simulink model "TASK7_kalman_filter"  (R2023b)
settings: Solver=VariableStepAuto  StartTime=0.0  StopTime=10  MaxStep=0.01  RelTol=1e-3  EnableMultiTasking=on
values from neighbouring files (symbols this model uses):
  b = 0.2    [TASK0_main_code.m]
  dphi0 = 0.1    [TASK0_main_code.m]
  dx0 = 0.01    [TASK0_main_code.m]
  g = 9.81    [TASK0_main_code.m]
  J_s = 1/3*m*l^2    (= 4.99725166667)    [TASK0_main_code.m]
  K = place(A_lin, B_lin, p)    [TASK0_main_code.m]
  KF = ss(A_lin-L*C_lin(2,:), [B_lin L], eye(4), 0*[B_lin L])    [TASK0_main_code.m]
  l = 3.11    [TASK0_main_code.m]
  m = 1.55    [TASK0_main_code.m]
  M = 7.87    [TASK0_main_code.m]
  noise_mean = 0    [TASK0_main_code.m]
  noise_sample_time = 0.001    [TASK0_main_code.m]
  noise_seed = 10000    [TASK0_main_code.m]
  phi0 = 0.05    [TASK0_main_code.m]
  sigma_wd = [ 1 , 0  , 0 , 0 ... (first row only)    [TASK0_main_code.m]
  sigma_wd2 = [ 1 , 0  , 0 , 0 ... (first row only)    [TASK0_main_code.m]
  sigma_wd3 = [ 10 , 0  , 0 , 0 ... (first row only)    [TASK0_main_code.m]
  sigma_wn = 0.1    [TASK0_main_code.m]
  x0 = -0.01    [TASK0_main_code.m]
libraries: dspinverses x3
settings Model: Creator=iklod_000  LastModifiedBy=piri
settings SolverCC: AlgebraicLoopSolver=TrustRegion
settings DataIOCC: ReturnWorkspaceOutputs=off
settings OptimizationCC: LifeSpan=inf
settings DebuggingCC: UnconnectedInputMsg=warning  UnconnectedOutputMsg=warning  UnconnectedLineMsg=warning  SFUnexpectedBacktrackingDiag=warning  SFNoUnconditionalDefaultTransitionDiag=warning  ArithmeticOperatorsInVariantConditions=warning
settings ModelReferenceCC: EnableRefExpFcnMdlSchedulingChecks=on
settings SFSimCC: SimUseLocalCustomCode=off  CustomCodeUndefinedFunction=UseInterfaceOnly
settings RTWCC: RTWUseLocalCustomCode=off
settings CodeAppCC: StateflowObjectComments=on
settings GRTTargetCC: TargetLangStandard=C89/C90 (ANSI)
settings ConfigComp: CovMetricSettings=dw  CovSaveCumulativeToWorkspaceVar=on  CovSaveSingleToWorkspaceVar=on  CovExternalEMLEnable=off

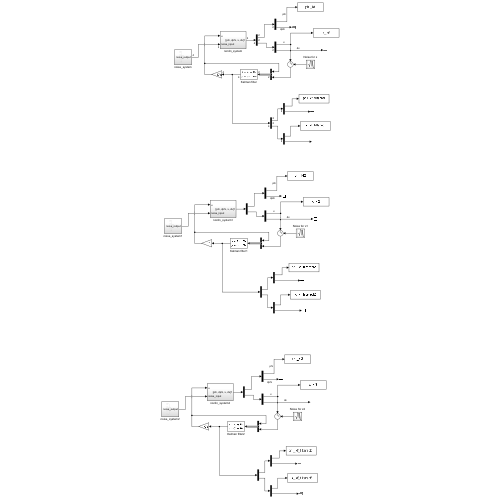
[thumbnail: Simulink's stored preview of the top-level diagram]
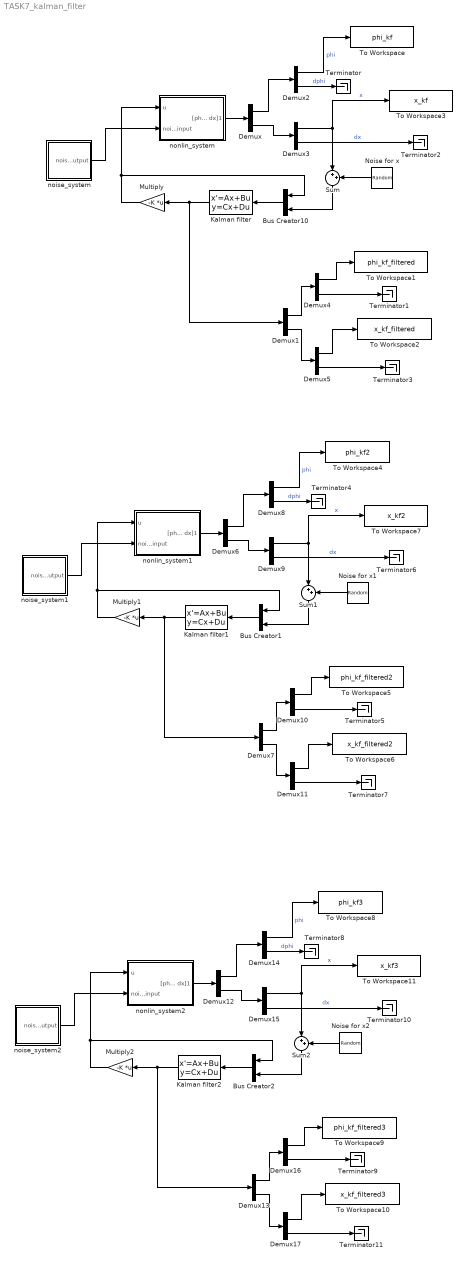
== system TASK7_kalman_filter ==
  Bus Creator1 : BusCreator  Inputs=2
  Bus Creator10 : BusCreator  Inputs=2
  Bus Creator2 : BusCreator  Inputs=2
  Demux{,1..17} (18 alike) : Demux  Outputs=2
  Kalman filter : StateSpace  A=KF.A  B=KF.B  C=KF.C  D=KF.D  InitialCondition=[phi0, dphi0, x0, dx0]
  Kalman filter1 : StateSpace  A=KF.A  B=KF.B  C=KF.C  D=KF.D  InitialCondition=[phi0, dphi0, x0, dx0]
  Kalman filter2 : StateSpace  A=KF.A  B=KF.B  C=KF.C  D=KF.D  InitialCondition=[phi0, dphi0, x0, dx0]
  Multiply : Gain  Gain=-K  Multiplication=Matrix(K*u)
  Multiply1 : Gain  Gain=-K  Multiplication=Matrix(K*u)
  Multiply2 : Gain  Gain=-K  Multiplication=Matrix(K*u)
  Noise for x : RandomNumber  Mean=noise_mean  Variance=sigma_wn  Seed=noise_seed  SampleTime=noise_sample_time
  Noise for x1 : RandomNumber  Mean=noise_mean  Variance=sigma_wn  Seed=noise_seed  SampleTime=noise_sample_time
  Noise for x2 : RandomNumber  Mean=noise_mean  Variance=sigma_wn  Seed=noise_seed  SampleTime=noise_sample_time
  Sum : Sum  Inputs=|++
  Sum1 : Sum  Inputs=|++
  Sum2 : Sum  Inputs=|++
  Terminator{,1..11} (12 alike) : Terminator
  To Workspace : ToWorkspace  VariableName=phi_kf  SaveFormat=Timeseries  SampleTime=-1
  To Workspace1 : ToWorkspace  VariableName=phi_kf_filtered  SaveFormat=Timeseries  SampleTime=-1
  To Workspace10 : ToWorkspace  VariableName=x_kf_filtered3  SaveFormat=Timeseries  SampleTime=-1
  To Workspace11 : ToWorkspace  VariableName=x_kf3  SaveFormat=Timeseries  SampleTime=-1
  To Workspace2 : ToWorkspace  VariableName=x_kf_filtered  SaveFormat=Timeseries  SampleTime=-1
  To Workspace3 : ToWorkspace  VariableName=x_kf  SaveFormat=Timeseries  SampleTime=-1
  To Workspace4 : ToWorkspace  VariableName=phi_kf2  SaveFormat=Timeseries  SampleTime=-1
  To Workspace5 : ToWorkspace  VariableName=phi_kf_filtered2  SaveFormat=Timeseries  SampleTime=-1
  To Workspace6 : ToWorkspace  VariableName=x_kf_filtered2  SaveFormat=Timeseries  SampleTime=-1
  To Workspace7 : ToWorkspace  VariableName=x_kf2  SaveFormat=Timeseries  SampleTime=-1
  To Workspace8 : ToWorkspace  VariableName=phi_kf3  SaveFormat=Timeseries  SampleTime=-1
  To Workspace9 : ToWorkspace  VariableName=phi_kf_filtered3  SaveFormat=Timeseries  SampleTime=-1
  noise_system : Subsystem
  noise_system1 : Subsystem
  noise_system2 : Subsystem
  nonlin_system : Subsystem
  nonlin_system1 : Subsystem
  nonlin_system2 : Subsystem
  wires:
  nonlin_system/1("[phi, dphi, x, dx]1") -> Demux/1
  Demux/1 -> Demux2/1
  Multiply/1 -> Bus Creator10/1, nonlin_system/1(u)
  Demux2/1 -> To Workspace/1  "phi"
  Demux2/2 -> Terminator/1  "dphi"
  Kalman filter/1 -> Demux1/1, Multiply/1
  Demux/2 -> Demux3/1
  Demux3/1 -> To Workspace3/1, Sum/1  "x"
  Noise for x/1 -> Sum/2
  Sum/1 -> Bus Creator10/2
  Bus Creator10/1 -> Kalman filter/1
  Demux3/2 -> Terminator2/1  "dx"
  Demux1/1 -> Demux4/1
  Demux1/2 -> Demux5/1
  Demux4/1 -> To Workspace1/1
  Demux4/2 -> Terminator1/1
  Demux5/1 -> To Workspace2/1
  Demux5/2 -> Terminator3/1
  noise_system/1(noise_output) -> nonlin_system/2(noise_input)
  Sum1/1 -> Bus Creator1/2
  Bus Creator1/1 -> Kalman filter1/1
  Demux9/2 -> Terminator6/1  "dx"
  Kalman filter1/1 -> Demux7/1, Multiply1/1
  Demux10/1 -> To Workspace5/1
  Demux7/2 -> Demux11/1
  Demux11/2 -> Terminator7/1
  Demux6/1 -> Demux8/1
  noise_system1/1(noise_output) -> nonlin_system1/2(noise_input)
  Noise for x1/1 -> Sum1/2
  Demux11/1 -> To Workspace6/1
  Demux10/2 -> Terminator5/1
  Demux9/1 -> To Workspace7/1, Sum1/1  "x"
  Demux6/2 -> Demux9/1
  Demux8/2 -> Terminator4/1  "dphi"
  nonlin_system1/1("[phi, dphi, x, dx]1") -> Demux6/1
  Demux7/1 -> Demux10/1
  Demux8/1 -> To Workspace4/1  "phi"
  Multiply1/1 -> Bus Creator1/1, nonlin_system1/1(u)
  Sum2/1 -> Bus Creator2/2
  Bus Creator2/1 -> Kalman filter2/1
  Demux15/2 -> Terminator10/1  "dx"
  Kalman filter2/1 -> Demux13/1, Multiply2/1
  Demux16/1 -> To Workspace9/1
  Demux13/2 -> Demux17/1
  Demux17/2 -> Terminator11/1
  Demux12/1 -> Demux14/1
  noise_system2/1(noise_output) -> nonlin_system2/2(noise_input)
  Noise for x2/1 -> Sum2/2
  Demux17/1 -> To Workspace10/1
  Demux16/2 -> Terminator9/1
  Demux15/1 -> To Workspace11/1, Sum2/1  "x"
  Demux12/2 -> Demux15/1
  Demux14/2 -> Terminator8/1  "dphi"
  nonlin_system2/1("[phi, dphi, x, dx]1") -> Demux12/1
  Demux13/1 -> Demux16/1
  Demux14/1 -> To Workspace8/1  "phi"
  Multiply2/1 -> Bus Creator2/1, nonlin_system2/1(u)

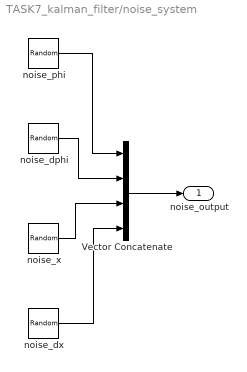
== system TASK7_kalman_filter/noise_system ==
  Vector Concatenate : Concatenate  NumInputs=4
  noise_dphi : RandomNumber  Mean=noise_mean  Variance=sigma_wd(2,2)  Seed=noise_seed  SampleTime=noise_sample_time
  noise_dx : RandomNumber  Mean=noise_mean  Variance=sigma_wd(4,4)  Seed=noise_seed  SampleTime=noise_sample_time
  noise_phi : RandomNumber  Mean=noise_mean  Variance=sigma_wd(1,1)  Seed=noise_seed  SampleTime=noise_sample_time
  noise_x : RandomNumber  Mean=noise_mean  Variance=sigma_wd(3,3)  Seed=noise_seed  SampleTime=noise_sample_time
  noise_output : Outport
  wires:
  Vector Concatenate/1 -> noise_output/1
  noise_phi/1 -> Vector Concatenate/1
  noise_dphi/1 -> Vector Concatenate/2
  noise_x/1 -> Vector Concatenate/3
  noise_dx/1 -> Vector Concatenate/4

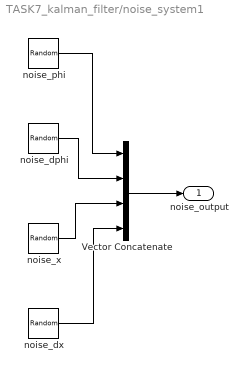
== system TASK7_kalman_filter/noise_system1 ==
  Vector Concatenate : Concatenate  NumInputs=4
  noise_dphi : RandomNumber  Mean=noise_mean  Variance=sigma_wd2(2,2)  Seed=noise_seed  SampleTime=noise_sample_time
  noise_dx : RandomNumber  Mean=noise_mean  Variance=sigma_wd2(4,4)  Seed=noise_seed  SampleTime=noise_sample_time
  noise_phi : RandomNumber  Mean=noise_mean  Variance=sigma_wd2(1,1)  Seed=noise_seed  SampleTime=noise_sample_time
  noise_x : RandomNumber  Mean=noise_mean  Variance=sigma_wd2(3,3)  Seed=noise_seed  SampleTime=noise_sample_time
  noise_output : Outport
  wires:
  Vector Concatenate/1 -> noise_output/1
  noise_phi/1 -> Vector Concatenate/1
  noise_dphi/1 -> Vector Concatenate/2
  noise_x/1 -> Vector Concatenate/3
  noise_dx/1 -> Vector Concatenate/4

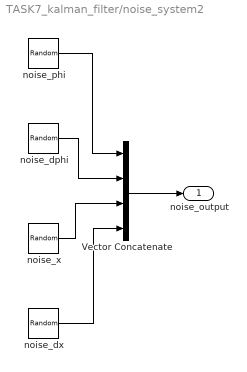
== system TASK7_kalman_filter/noise_system2 ==
  Vector Concatenate : Concatenate  NumInputs=4
  noise_dphi : RandomNumber  Mean=noise_mean  Variance=sigma_wd3(2,2)  Seed=noise_seed  SampleTime=noise_sample_time
  noise_dx : RandomNumber  Mean=noise_mean  Variance=sigma_wd3(4,4)  Seed=noise_seed  SampleTime=noise_sample_time
  noise_phi : RandomNumber  Mean=noise_mean  Variance=sigma_wd3(1,1)  Seed=noise_seed  SampleTime=noise_sample_time
  noise_x : RandomNumber  Mean=noise_mean  Variance=sigma_wd3(3,3)  Seed=noise_seed  SampleTime=noise_sample_time
  noise_output : Outport
  wires:
  Vector Concatenate/1 -> noise_output/1
  noise_phi/1 -> Vector Concatenate/1
  noise_dphi/1 -> Vector Concatenate/2
  noise_x/1 -> Vector Concatenate/3
  noise_dx/1 -> Vector Concatenate/4

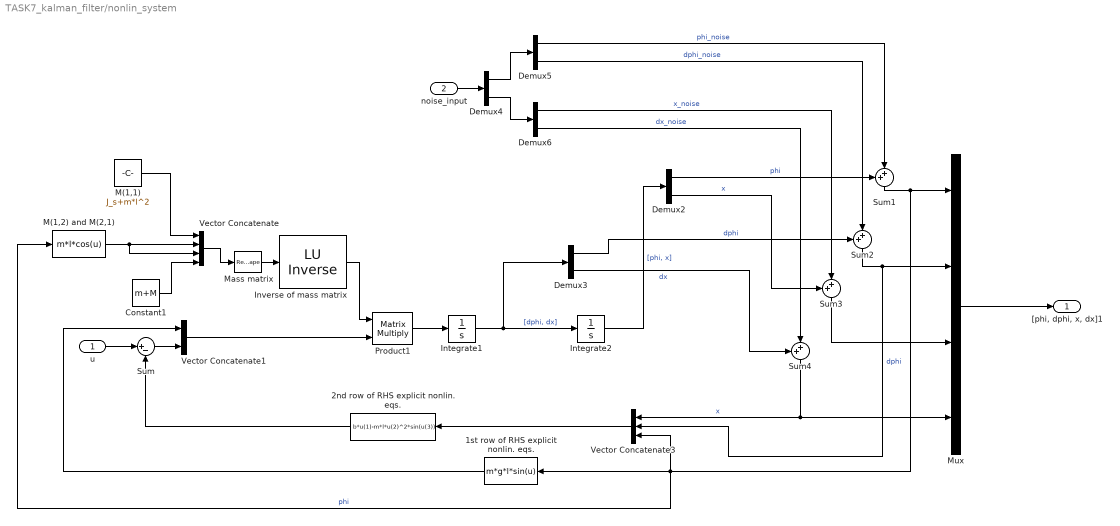
== system TASK7_kalman_filter/nonlin_system ==
  u : Inport
  noise_input : Inport  Port=2
  1st row of RHS explicit nonlin. eqs. : Fcn  Expr=m*g*l*sin(u)
  2nd row of RHS explicit nonlin. eqs. : Fcn  Expr=b*u(1)-m*l*u(2)^2*sin(u(3))
  Constant1 : Constant  Value=m+M
  Demux{2..6} (5 alike) : Demux  Outputs=2
  Integrate1 : Integrator  InitialCondition=[dphi0; dx0]
  Integrate2 : Integrator  InitialCondition=[phi0; x0]
  Inverse of mass matrix : dspinverses/ LU Inverse
  M(1,1) : Constant  Value=J_s+m*l^2
  M(1,2) and M(2,1) : Fcn  Expr=m*l*cos(u)
  Mass matrix : Reshape  OutputDimensionality=Customize  OutputDimensions=[2,2]
  Mux : Mux
  Product1 : Product  Multiplication=Matrix(*)
  Sum : Sum  Inputs=|+-
  Sum{1..4} (4 alike) : Sum  Inputs=++|
  Vector Concatenate : Concatenate  NumInputs=4
  Vector Concatenate1 : Concatenate
  Vector Concatenate3 : Concatenate  NumInputs=3
  "[phi, dphi, x, dx]1" : Outport
  wires:
  Mass matrix/1 -> Inverse of mass matrix/1
  u/1 -> Sum/1
  Constant1/1 -> Vector Concatenate/4
  Inverse of mass matrix/1 -> Product1/1
  Vector Concatenate3/1 -> 2nd row of RHS explicit nonlin. eqs./1
  Vector Concatenate1/1 -> Product1/2
  1st row of RHS explicit nonlin. eqs./1 -> Vector Concatenate1/1
  Sum/1 -> Vector Concatenate1/2
  2nd row of RHS explicit nonlin. eqs./1 -> Sum/2
  Vector Concatenate/1 -> Mass matrix/1
  M(1,1)/1 -> Vector Concatenate/1
  M(1,2) and M(2,1)/1 -> Vector Concatenate/3, Vector Concatenate/2
  Product1/1 -> Integrate1/1
  Integrate1/1 -> Demux3/1, Integrate2/1  "[dphi, dx]"
  Integrate2/1 -> Demux2/1  "[phi, x]"
  Sum1/1 -> 1st row of RHS explicit nonlin. eqs./1, Vector Concatenate3/3, M(1,2) and M(2,1)/1, Mux/1  "phi"
  Mux/1 -> "[phi, dphi, x, dx]1"/1
  noise_input/1 -> Demux4/1
  Demux4/1 -> Demux5/1
  Demux4/2 -> Demux6/1
  Demux5/1 -> Sum1/2  "phi_noise"
  Demux5/2 -> Sum2/2  "dphi_noise"
  Demux6/1 -> Sum3/2  "x_noise"
  Demux6/2 -> Sum4/2  "dx_noise"
  Demux3/1 -> Sum2/1  "dphi"
  Demux3/2 -> Sum4/1  "dx"
  Demux2/1 -> Sum1/1  "phi"
  Demux2/2 -> Sum3/1  "x"
  Sum2/1 -> Vector Concatenate3/2, Mux/2  "dphi"
  Sum3/1 -> Mux/3
  Sum4/1 -> Vector Concatenate3/1, Mux/4  "x"

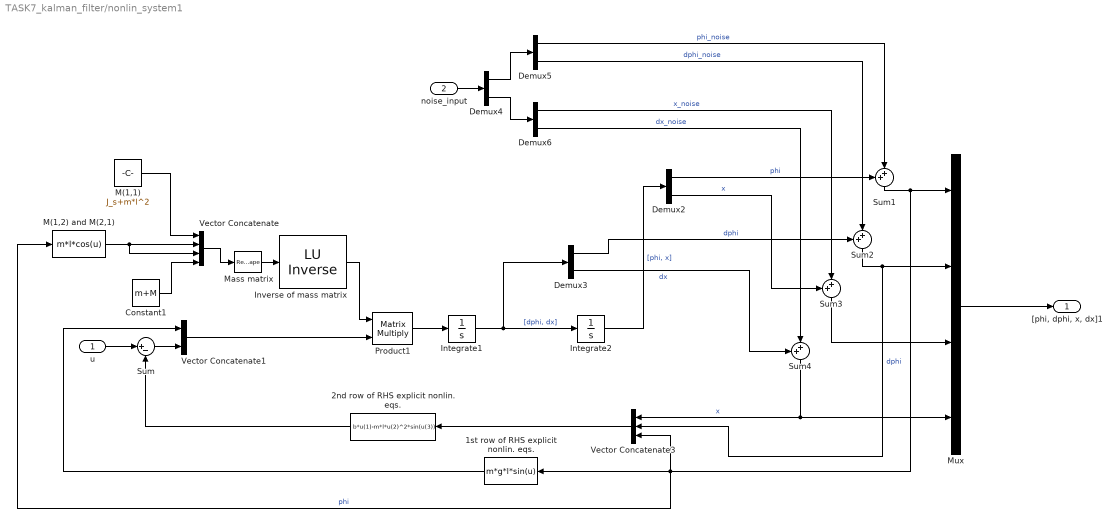
== system TASK7_kalman_filter/nonlin_system1 ==
  u : Inport
  noise_input : Inport  Port=2
  1st row of RHS explicit nonlin. eqs. : Fcn  Expr=m*g*l*sin(u)
  2nd row of RHS explicit nonlin. eqs. : Fcn  Expr=b*u(1)-m*l*u(2)^2*sin(u(3))
  Constant1 : Constant  Value=m+M
  Demux{2..6} (5 alike) : Demux  Outputs=2
  Integrate1 : Integrator  InitialCondition=[dphi0; dx0]
  Integrate2 : Integrator  InitialCondition=[phi0; x0]
  Inverse of mass matrix : dspinverses/ LU Inverse
  M(1,1) : Constant  Value=J_s+m*l^2
  M(1,2) and M(2,1) : Fcn  Expr=m*l*cos(u)
  Mass matrix : Reshape  OutputDimensionality=Customize  OutputDimensions=[2,2]
  Mux : Mux
  Product1 : Product  Multiplication=Matrix(*)
  Sum : Sum  Inputs=|+-
  Sum{1..4} (4 alike) : Sum  Inputs=++|
  Vector Concatenate : Concatenate  NumInputs=4
  Vector Concatenate1 : Concatenate
  Vector Concatenate3 : Concatenate  NumInputs=3
  "[phi, dphi, x, dx]1" : Outport
  wires:
  Mass matrix/1 -> Inverse of mass matrix/1
  u/1 -> Sum/1
  Constant1/1 -> Vector Concatenate/4
  Inverse of mass matrix/1 -> Product1/1
  Vector Concatenate3/1 -> 2nd row of RHS explicit nonlin. eqs./1
  Vector Concatenate1/1 -> Product1/2
  1st row of RHS explicit nonlin. eqs./1 -> Vector Concatenate1/1
  Sum/1 -> Vector Concatenate1/2
  2nd row of RHS explicit nonlin. eqs./1 -> Sum/2
  Vector Concatenate/1 -> Mass matrix/1
  M(1,1)/1 -> Vector Concatenate/1
  M(1,2) and M(2,1)/1 -> Vector Concatenate/3, Vector Concatenate/2
  Product1/1 -> Integrate1/1
  Integrate1/1 -> Demux3/1, Integrate2/1  "[dphi, dx]"
  Integrate2/1 -> Demux2/1  "[phi, x]"
  Sum1/1 -> 1st row of RHS explicit nonlin. eqs./1, Vector Concatenate3/3, M(1,2) and M(2,1)/1, Mux/1  "phi"
  Mux/1 -> "[phi, dphi, x, dx]1"/1
  noise_input/1 -> Demux4/1
  Demux4/1 -> Demux5/1
  Demux4/2 -> Demux6/1
  Demux5/1 -> Sum1/2  "phi_noise"
  Demux5/2 -> Sum2/2  "dphi_noise"
  Demux6/1 -> Sum3/2  "x_noise"
  Demux6/2 -> Sum4/2  "dx_noise"
  Demux3/1 -> Sum2/1  "dphi"
  Demux3/2 -> Sum4/1  "dx"
  Demux2/1 -> Sum1/1  "phi"
  Demux2/2 -> Sum3/1  "x"
  Sum2/1 -> Vector Concatenate3/2, Mux/2  "dphi"
  Sum3/1 -> Mux/3
  Sum4/1 -> Vector Concatenate3/1, Mux/4  "x"

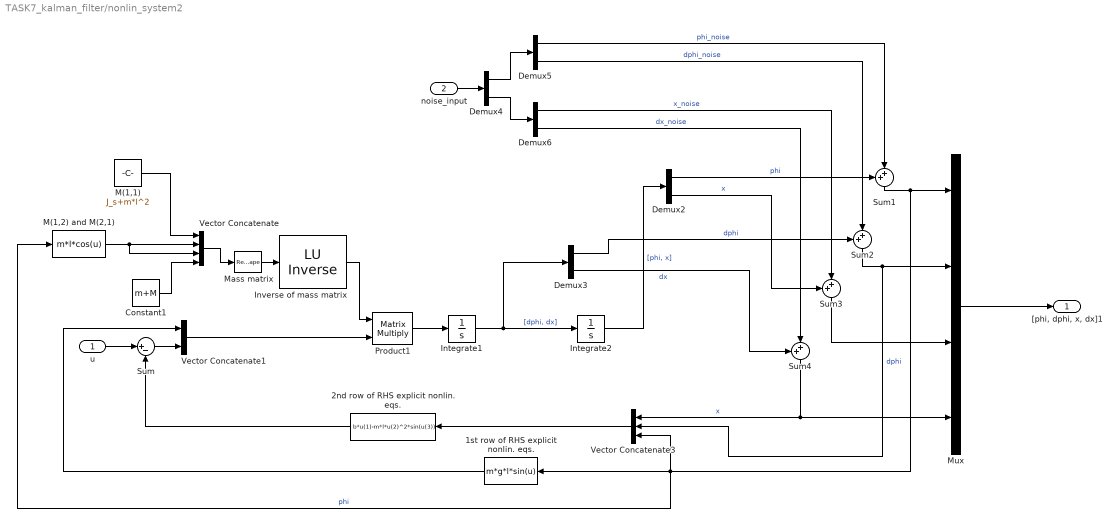
== system TASK7_kalman_filter/nonlin_system2 ==
  u : Inport
  noise_input : Inport  Port=2
  1st row of RHS explicit nonlin. eqs. : Fcn  Expr=m*g*l*sin(u)
  2nd row of RHS explicit nonlin. eqs. : Fcn  Expr=b*u(1)-m*l*u(2)^2*sin(u(3))
  Constant1 : Constant  Value=m+M
  Demux{2..6} (5 alike) : Demux  Outputs=2
  Integrate1 : Integrator  InitialCondition=[dphi0; dx0]
  Integrate2 : Integrator  InitialCondition=[phi0; x0]
  Inverse of mass matrix : dspinverses/ LU Inverse
  M(1,1) : Constant  Value=J_s+m*l^2
  M(1,2) and M(2,1) : Fcn  Expr=m*l*cos(u)
  Mass matrix : Reshape  OutputDimensionality=Customize  OutputDimensions=[2,2]
  Mux : Mux
  Product1 : Product  Multiplication=Matrix(*)
  Sum : Sum  Inputs=|+-
  Sum{1..4} (4 alike) : Sum  Inputs=++|
  Vector Concatenate : Concatenate  NumInputs=4
  Vector Concatenate1 : Concatenate
  Vector Concatenate3 : Concatenate  NumInputs=3
  "[phi, dphi, x, dx]1" : Outport
  wires:
  Mass matrix/1 -> Inverse of mass matrix/1
  u/1 -> Sum/1
  Constant1/1 -> Vector Concatenate/4
  Inverse of mass matrix/1 -> Product1/1
  Vector Concatenate3/1 -> 2nd row of RHS explicit nonlin. eqs./1
  Vector Concatenate1/1 -> Product1/2
  1st row of RHS explicit nonlin. eqs./1 -> Vector Concatenate1/1
  Sum/1 -> Vector Concatenate1/2
  2nd row of RHS explicit nonlin. eqs./1 -> Sum/2
  Vector Concatenate/1 -> Mass matrix/1
  M(1,1)/1 -> Vector Concatenate/1
  M(1,2) and M(2,1)/1 -> Vector Concatenate/3, Vector Concatenate/2
  Product1/1 -> Integrate1/1
  Integrate1/1 -> Demux3/1, Integrate2/1  "[dphi, dx]"
  Integrate2/1 -> Demux2/1  "[phi, x]"
  Sum1/1 -> 1st row of RHS explicit nonlin. eqs./1, Vector Concatenate3/3, M(1,2) and M(2,1)/1, Mux/1  "phi"
  Mux/1 -> "[phi, dphi, x, dx]1"/1
  noise_input/1 -> Demux4/1
  Demux4/1 -> Demux5/1
  Demux4/2 -> Demux6/1
  Demux5/1 -> Sum1/2  "phi_noise"
  Demux5/2 -> Sum2/2  "dphi_noise"
  Demux6/1 -> Sum3/2  "x_noise"
  Demux6/2 -> Sum4/2  "dx_noise"
  Demux3/1 -> Sum2/1  "dphi"
  Demux3/2 -> Sum4/1  "dx"
  Demux2/1 -> Sum1/1  "phi"
  Demux2/2 -> Sum3/1  "x"
  Sum2/1 -> Vector Concatenate3/2, Mux/2  "dphi"
  Sum3/1 -> Mux/3
  Sum4/1 -> Vector Concatenate3/1, Mux/4  "x"
